simulink model "simul_RST"  (R2023b)
settings: Solver=VariableStepAuto  StartTime=0.0  StopTime=10.0  RelTol=1e-3
values from neighbouring files (symbols this model uses):
  R = SR(nS+1:end)    [rst.m]    (also in rst_int.m; script2_waterloo.m = x(4:5); untitled.m)
  S = SR(1:nS)    [rst.m]    (also in rst_int.m = S'; script2_waterloo.m = x(1:3); untitled.m)
  T = t(2)-t(1)    [frecventa.m]    (also in rst.m = sum(P)/sum(B); rst_int.m = sum(P)/sum(B); script2_waterloo.m = sum(P)/sum(B); untitled.m = sum(P)/sum(B))
settings Model: Creator=wombelbat  LastModifiedBy=wombelbat

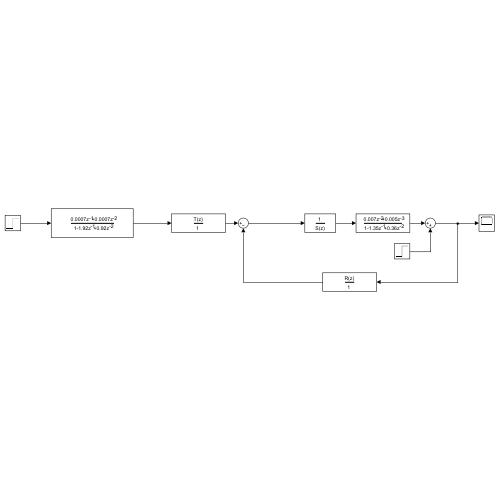
[thumbnail: Simulink's stored preview of the top-level diagram]
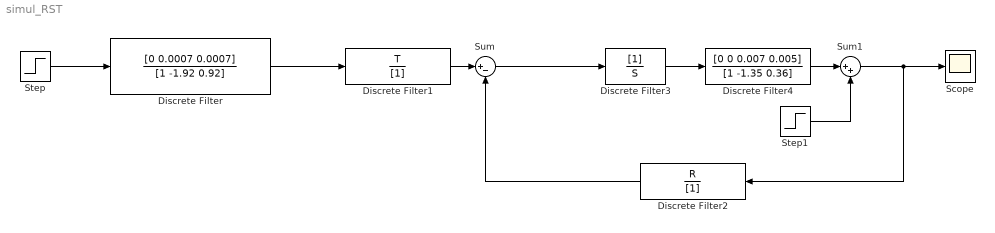
== system simul_RST ==
  Discrete Filter : DiscreteFilter  Numerator=[0 0.0007 0.0007]  Denominator=[1 -1.92 0.92]
  Discrete Filter1 : DiscreteFilter  Numerator=T  Denominator=[1]
  Discrete Filter2 : DiscreteFilter  Numerator=R  Denominator=[1]
  Discrete Filter3 : DiscreteFilter  Denominator=S
  Discrete Filter4 : DiscreteFilter  Numerator=[0 0 0.007 0.005]  Denominator=[1 -1.35 0.36]
  Scope : Scope
  Step : Step  Time=0  After=50  SampleTime=0.1
  Step1 : Step  Time=0  After=0  SampleTime=0.1
  Sum : Sum  Inputs=|+-
  Sum1 : Sum  Inputs=|++
  wires:
  Step/1 -> Discrete Filter/1
  Sum/1 -> Discrete Filter3/1
  Discrete Filter2/1 -> Sum/2
  Discrete Filter4/1 -> Sum1/1
  Sum1/1 -> Discrete Filter2/1, Scope/1
  Step1/1 -> Sum1/2
  Discrete Filter3/1 -> Discrete Filter4/1
  Discrete Filter1/1 -> Sum/1
  Discrete Filter/1 -> Discrete Filter1/1
